simulink model "VehicleDynamicsModel"  (R2018a)
settings: Solver=ode15s  StartTime=0.0  StopTime=12  FixedStep=0.01  RelTol=1e-2  EnableMultiTasking=on
PreLoadFcn:
  | PowerTrain_14DOF_ini
StopFcn:
  | AfterSim
undefined symbols (not defined in the file): AccelCmd2TrqCmd, Chasis, GearRatio, Motor, Motor_J, Motor_RotorDamping, VEH, X, Y, Z
libraries: sm_lib x186, autolibutils x40, nesl_utility x23, vehdynlibtire x4, fuzblock x3, sharedtransform x2, autolibmappedmotorcommon x2, vehdynlibeom x1, vehdynlibsuspension x1, simulink x1, vehdynlibsteering x1
(part 1 of 11)
settings Model: SimulationMode=accelerator  ExtModeTrigDuration=100  Creator=rjackey  LastModifiedBy=Administrator
settings DataIOCC: ExternalInput=[Throttle.Time Throttle.Data Brake.Data]  LimitDataPoints=on  SaveFormat=StructureWithTime  SaveOutput=off  DSMLogging=off  SaveTime=off  StateSaveName=tmp_raccel_xout  OutputSaveName=out
settings OptimizationCC: DefaultUnderspecifiedDataType=single  ExpressionDepthLimit=2147483647  EfficientMapNaN2IntZero=off  LifeSpan=inf
settings DebuggingCC: UnderspecifiedInitializationDetection=Classic  MergeDetectMultiDrivingBlocksExec=none  SolverPrmCheckMsg=warning  UnnecessaryDatatypeConvMsg=warning  FcnCallInpInsideContextMsg=warning  StateNameClashWarn=warning  SFUnexpectedBacktrackingDiag=warning  SFNoUnconditionalDefaultTransitionDiag=warning  SFExecutionAtInitializationDiag=none
settings HardwareCC: ProdBitPerPointer=32  ProdBitPerSizeT=32  ProdBitPerPtrDiffT=32  ProdLargestAtomicFloat=None  ProdIntDivRoundTo=Undefined  ProdEndianess=Unspecified  ProdWordSize=32  ProdHWDeviceType=32-bit Generic  TargetBitPerPointer=64  TargetBitPerSizeT=64  TargetBitPerPtrDiffT=64  TargetLongLongMode=on  TargetIntDivRoundTo=Zero  TargetEndianess=LittleEndian  TargetWordSize=64  TargetHWDeviceType=MATLAB Host  ProdEqTarget=off
settings ModelReferenceCC: PropagateSignalLabelsOutOfModel=off
settings RTWCC: SystemTargetFile=raccel.tlc  TemplateMakefile=raccel_default_tmf  RTWVerbose=off  RTWUseSimCustomCode=on
settings CodeAppCC: GenerateComments=off  MaxIdLength=128  MangleLength=10
settings RaccelTargetCC: GeneratePreprocessorConditionals=Use local settings  MultiInstanceERTCode=off  ENABLE_SLEXEC_SSBRIDGE=1  RTWCAPIParams=on
settings ConfigComp: CovScope=ReferencedModels  CovIncludeTopModel=off  CovMetricSettings=dw  CovHtmlReporting=on  CovSaveCumulativeToWorkspaceVar=on  CovSaveSingleToWorkspaceVar=on  CovExternalEMLEnable=off
settings SimscapeCC: SimscapeNormalizeSystem=off
settings ExplorerConfigSet: SimMechanicsOpenEditorOnUpdate=off

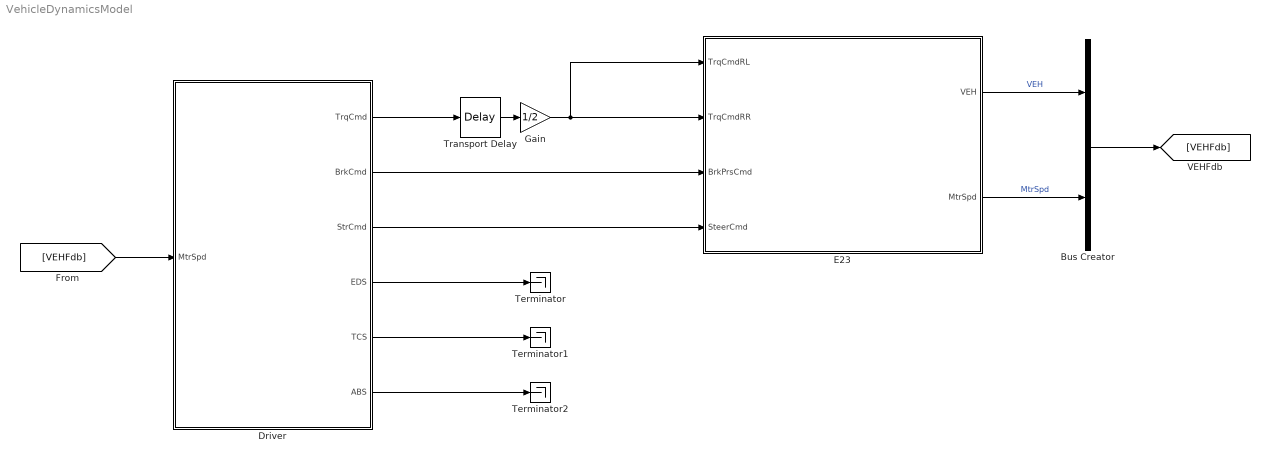
== system VehicleDynamicsModel ==
  Bus Creator : BusCreator  Inputs=2
  Driver : Subsystem
      mask Display: image('Driver.JPEG');
  E23 : Subsystem
      mask Display: image('E2314DOF2.jpg')
  Gain : Gain  Gain=1/2
  Terminator : Terminator
  Terminator1 : Terminator
  Terminator2 : Terminator
  Transport Delay : TransportDelay  DelayTime=0.1
  wires:
  Driver/3(StrCmd) -> E23/4(SteerCmd)
  Driver/2(BrkCmd) -> E23/3(BrkPrsCmd)
  E23/2(MtrSpd) -> Bus Creator/2  "MtrSpd"
  E23/1(VEH) -> Bus Creator/1  "VEH"
  Bus Creator/1 -> [VEHFdb]
  [VEHFdb] -> Driver/1(MtrSpd)
  Driver/1(TrqCmd) -> Transport Delay/1
  Gain/1 -> E23/2(TrqCmdRR), E23/1(TrqCmdRL)
  Transport Delay/1 -> Gain/1
  Driver/4(EDS) -> Terminator/1
  Driver/5(TCS) -> Terminator1/1
  Driver/6(ABS) -> Terminator2/1

== system VehicleDynamicsModel/Driver ==
  MtrSpd : Inport
  AccCmdGenerate : Subsystem
  Accel : Subsystem
  BrkCmdGenerate : Subsystem
  Bus Selector : BusSelector  OutputSignals=MtrSpd.MtrSpdRL,MtrSpd.MtrSpdRR
  Constant{1,5..7} (4 alike) : Constant  Value=0
  Mux : Mux
  Saturation : Saturate  UpperLimit=1  LowerLimit=0
  StrCmdGenerate : Subsystem
  Terminator3 : Terminator
  TrqCmd : Outport
  BrkCmd : Outport  Port=2
  StrCmd : Outport  Port=3
  EDS : Outport  Port=4
  TCS : Outport  Port=5
  ABS : Outport  Port=6
  wires:
  Saturation/1 -> Accel/3(AccelCmd)
  Constant5/1 -> EDS/1
  MtrSpd/1 -> Bus Selector/1
  Constant1/1 -> Mux/2, Mux/1, Mux/4, Mux/3
  Constant6/1 -> TCS/1
  Accel/1(TrqCmd) -> TrqCmd/1
  Constant7/1 -> ABS/1
  Bus Selector/2 -> Accel/2(MtrSpdRR)  "<MtrSpdRR>"
  Bus Selector/1 -> Accel/1(MtrSpdRL)  "<MtrSpdRL>"
  Mux/1 -> BrkCmd/1
  BrkCmdGenerate/1(BrkCmd) -> Terminator3/1  "BrkCmd"
  AccCmdGenerate/1(AccCmd) -> Saturation/1  "AccCmd"
  StrCmdGenerate/1(StrCmd) -> StrCmd/1  "StrCmd"

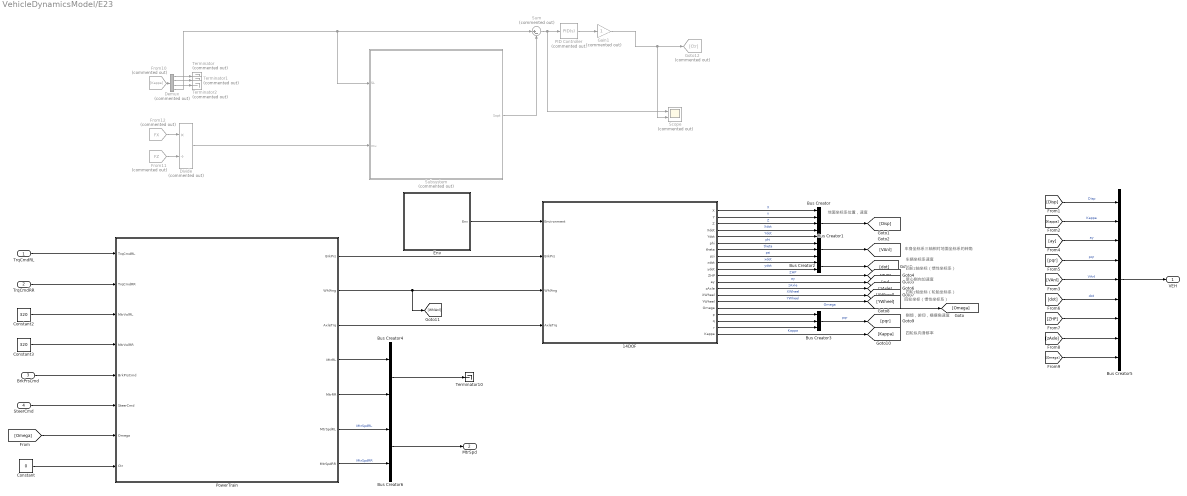
== system VehicleDynamicsModel/E23 ==
  note: 侧倾，俯仰，横摆角速度
  note: 四轮坐标（惯性坐标系）
  note: 质心侧向加速度
  note: 四轮z轴坐标（惯性坐标系）
  note: 车身坐标系三轴相对地面坐标系的转角
  note: 地面坐标系位置，速度
  note: 车辆坐标系速度
  note: 四轮z轴坐标（轮胎坐标系）
  note: 四轮纵向滑移率
  TrqCmdRL : Inport
  TrqCmdRR : Inport  Port=2
  BrkPrsCmd : Inport  Port=3
  SteerCmd : Inport  Port=4
  14DOF : Subsystem
      mask Display: image('E2314DOF.jpg')
  Bus Creator : BusCreator  Inputs=5
  Bus Creator1 : BusCreator  Inputs=3
  Bus Creator2 : BusCreator  Inputs=2
  Bus Creator3 : BusCreator  Inputs=3
  Bus Creator4 : BusCreator  Inputs=2
  Bus Creator5 : BusCreator  Inputs=9
  Bus Creator6 : BusCreator  Inputs=2
  Constant : Constant  Value=0
  Constant2 : Constant  Value=320
  Constant3 : Constant  Value=320
  Demux : Demux  Commented=on
  Divide : Product  Commented=on  Inputs=*/
  Env : Subsystem
      mask Display: image('Env.jpg')
  From10 : From  Commented=on  GotoTag=Kappa
  From11 : From  Commented=on  GotoTag=FZ  TagVisibility=global
  From12 : From  Commented=on  GotoTag=FX  TagVisibility=global
  Gain1 : Gain  Commented=on
  Goto12 : Goto  Commented=on  GotoTag=Ctr
  PID Controller : simulink/Continuous/PID Controller  Commented=on  Controller=PID  TimeDomain=Continuous-time  SampleTime=-1  IntegratorMethod=Forward Euler  FilterMethod=Forward Euler  Form=Parallel  UseFilter=on  ControllerParametersSource=internal  P=500  I=20  D=0  N=100  InitialConditionSource=internal  InitialConditionForIntegrator=0  InitialConditionForFilter=0  ExternalReset=none  LimitOutput=off  UpperSaturationLimit=inf  LowerSaturationLimit=-inf  LinearizeAsGain=on  AntiWindupMode=none  Kb=1  TrackingMode=off  Kt=1  PParamMin=[]  PParamMax=[]  IParamMin=[]  IParamMax=[]  DParamMin=[]  DParamMax=[]  NParamMin=[]  NParamMax=[]  KbParamMin=[]  KbParamMax=[]  KtParamMin=[]  KtParamMax=[]  POutMin=[]  POutMax=[]  IOutMin=[]  IOutMax=[]  DOutMin=[]  DOutMax=[]  NOutMin=[]  NOutMax=[]  KbOutMin=[]  KbOutMax=[]  KtOutMin=[]  KtOutMax=[]  IntegratorOutMin=[]  IntegratorOutMax=[]  FilterOutMin=[]  FilterOutMax=[]  SumOutMin=[]  SumOutMax=[]  SumI1OutMin=[]  SumI1OutMax=[]  SumI2OutMin=[]  SumI2OutMax=[]  SumI3OutMin=[]  SumI3OutMax=[]  SumDOutMin=[]  SumDOutMax=[]  SaturationOutMin=[]  SaturationOutMax=[]  IntegratorContinuousStateAttributes=''  IntegratorStateMustResolveToSignalObject=off  IntegratorRTWStateStorageClass=Auto  FilterContinuousStateAttributes=''  FilterStateMustResolveToSignalObject=off  FilterRTWStateStorageClass=Auto  DifferentiatorICPrevScaledInput=0  DifferentiatorOutMin=[]  DifferentiatorOutMax=[]  FilterDiffOutCoefMin=[]  FilterDiffOutCoefMax=[]  SumDenOutMin=[]  SumDenOutMax=[]  SumNumOutMin=[]  SumNumOutMax=[]  ReciprocalOutMin=[]  ReciprocalOutMax=[]  DivideOutMin=[]  DivideOutMax=[]  TunerSelectOption=Transfer Function Based (PID Tuner App)
  PowerTrain : Subsystem
      mask Display: image('PowerTrain.jpg')
  Scope : Scope  Commented=on  NumInputPorts=2
  Subsystem : Subsystem  Commented=on
  Sum : Sum  Commented=on  Inputs=|+-
  Terminator : Terminator  Commented=on
  Terminator1 : Terminator  Commented=on
  Terminator10 : Terminator
  Terminator2 : Terminator  Commented=on
  VEH : Outport
  MtrSpd : Outport  Port=2
  wires:
  Bus Creator3/1 -> [pqr]  "pqr"
  14DOF/20(Kappa) -> [Kappa]  "Kappa"
  14DOF/15(YWheel) -> [YWheel]  "YWheel"
  14DOF/9(xdot) -> Bus Creator2/1  "xdot"
  [VAnl] -> Bus Creator5/5  "VAnl"
  PowerTrain/3(AxleTrq) -> 14DOF/4(AxleTrq)
  Bus Creator1/1 -> [VAnl]
  Bus Creator5/1 -> VEH/1
  14DOF/18(q) -> Bus Creator3/2
  Bus Creator/1 -> [Disp]
  [dot] -> Bus Creator5/6  "dot"
  14DOF/12(ay) -> [ay]  "ay"
  [pqr] -> Bus Creator5/4  "pqr"
  Bus Creator2/1 -> [dot]
  14DOF/14(XWheel) -> [XWheel]  "XWheel"
  PowerTrain/2(WhlAng) -> [WhlAnl], 14DOF/3(WhlAng)
  14DOF/11(ZHP) -> [ZHP]  "ZHP"
  TrqCmdRR/1 -> PowerTrain/2(TrqCmdRR)
  14DOF/7(theta) -> Bus Creator1/2  "theta"
  14DOF/16(Omega) -> [Omega]  "Omega"
  14DOF/1(X) -> Bus Creator/1  "X"
  14DOF/19(r) -> Bus Creator3/3
  Env/1(Env) -> 14DOF/1(Environment)
  14DOF/17(p) -> Bus Creator3/1
  14DOF/2(Y) -> Bus Creator/2  "Y"
  14DOF/3(Z) -> Bus Creator/3  "Z"
  [Disp] -> Bus Creator5/1  "Disp"
  PowerTrain/1(BrkPrs) -> 14DOF/2(BrkPrs)
  14DOF/5(Ydot) -> Bus Creator/5  "Ydot"
  14DOF/4(Xdot) -> Bus Creator/4  "Xdot"
  14DOF/6(phi) -> Bus Creator1/1  "phi"
  14DOF/10(ydot) -> Bus Creator2/2  "ydot"
  SteerCmd/1 -> PowerTrain/6(SteerCmd)
  PowerTrain/4(MtrRL) -> Bus Creator4/1
  Bus Creator4/1 -> Terminator10/1
  TrqCmdRL/1 -> PowerTrain/1(TrqCmdRL)
  Constant2/1 -> PowerTrain/3(MtrVolRL)
  Constant3/1 -> PowerTrain/4(MtrVolRR)
  BrkPrsCmd/1 -> PowerTrain/5(BrkPrsCmd)
  PowerTrain/5(MtrRR) -> Bus Creator4/2
  14DOF/8(psi) -> Bus Creator1/3  "psi"
  [Omega] -> PowerTrain/7(Omega)
  [Kappa] -> Bus Creator5/2  "Kappa"
  [ay] -> Bus Creator5/3  "ay"
  14DOF/13(zAxle) -> [zAxle]  "zAxle"
  [ZHP] -> Bus Creator5/7
  [zAxle] -> Bus Creator5/8
  [Omega] -> Bus Creator5/9
  PowerTrain/6(MtrSpdRL) -> Bus Creator6/1  "MtrSpdRL"
  PowerTrain/7(MtrSpdRR) -> Bus Creator6/2  "MtrSpdRR"
  Bus Creator6/1 -> MtrSpd/1
  Demux/4 -> Subsystem/1(SL), Sum/1
  Gain1/1 -> Scope/2, Goto12/1
  Subsystem/1(Sopt) -> Sum/2
  Sum/1 -> Scope/1, PID Controller/1
  Divide/1 -> Subsystem/2(mu)
  PID Controller/1 -> Gain1/1
  From10/1 -> Demux/1
  Demux/1 -> Terminator/1
  Demux/2 -> Terminator1/1
  Demux/3 -> Terminator2/1
  From12/1 -> Divide/1
  From11/1 -> Divide/2
  Constant/1 -> PowerTrain/8(Ctr)

== system VehicleDynamicsModel/Driver/AccCmdGenerate ==
  Clock : Clock
  Constant : Constant
  Constant1 : Constant  Value=0
  Constant2 : Constant  Value=0.1
  Switch : Switch  Criteria=u2 > Threshold  Threshold=4
  Switch1 : Switch  Criteria=u2 > Threshold  Threshold=8
  AccCmd : Outport
  wires:
  Constant1/1 -> Switch/1
  Switch1/1 -> AccCmd/1
  Clock/1 -> Switch1/2, Switch/2
  Constant2/1 -> Switch1/1
  Switch/1 -> Switch1/3
  Constant/1 -> Switch/3

== system VehicleDynamicsModel/Driver/Accel ==
  MtrSpdRL : Inport
  MtrSpdRR : Inport  Port=2
  AccelCmd : Inport  Port=3
  Add : Sum
  LookupTable : Lookup_n-D  BreakpointsForDimension1=AccelCmd2TrqCmd.Motor_n  BreakpointsForDimension2=fliplr(AccelCmd2TrqCmd.AccelCmd)  Table=fliplr(AccelCmd2TrqCmd.TrqCmd)  InternalRulePriority=Speed  RndMeth=Simplest  InputSameDT=on
  LookupTable1 : Lookup_n-D  BreakpointsForDimension1=AccelCmd2TrqCmd.Motor_n  BreakpointsForDimension2=fliplr(AccelCmd2TrqCmd.AccelCmd)  Table=fliplr(AccelCmd2TrqCmd.TrqCmd)  InternalRulePriority=Speed  RndMeth=Simplest  InputSameDT=on
  TrqCmd : Outport
  wires:
  LookupTable/1 -> Add/1
  MtrSpdRL/1 -> LookupTable/1
  MtrSpdRR/1 -> LookupTable1/1
  AccelCmd/1 -> LookupTable1/2, LookupTable/2
  LookupTable1/1 -> Add/2
  Add/1 -> TrqCmd/1

== system VehicleDynamicsModel/Driver/BrkCmdGenerate ==
  Clock : Clock
  Constant : Constant  Value=0
  Constant1 : Constant  Value=0.6
  Constant2 : Constant  Value=0
  Switch : Switch  Criteria=u2 > Threshold  Threshold=5
  Switch1 : Switch  Criteria=u2 > Threshold  Threshold=5.5
  BrkCmd : Outport
  wires:
  Constant/1 -> Switch/3
  Switch/1 -> Switch1/3
  Constant2/1 -> Switch1/1
  Clock/1 -> Switch/2, Switch1/2
  Switch1/1 -> BrkCmd/1
  Constant1/1 -> Switch/1

== system VehicleDynamicsModel/Driver/StrCmdGenerate ==
  Sine Wave : Sin  Amplitude=0.6  Frequency=3.1415926/3  SampleTime=0
  Transport Delay : TransportDelay  DelayTime=6
  StrCmd : Outport
  wires:
  Transport Delay/1 -> StrCmd/1
  Sine Wave/1 -> Transport Delay/1

== system VehicleDynamicsModel/E23/14DOF ==
  note: 双电机后驱
  Environment : Inport
  BrkPrs : Inport  Port=2
  WhlAng : Inport  Port=3
  AxleTrq : Inport  Port=4
  14DOF : Subsystem
      mask Display: image('E2314DOF2.jpg')
  Bus Creator : BusCreator  Inputs=4
  Bus Selector : BusSelector  OutputSignals=Wind,Gnd,mu
  Bus Selector2 : BusSelector  OutputSignals=p,q,r
  Demux : Demux
  X : Outport
  Y : Outport  Port=2
  Z : Outport  Port=3
  Xdot : Outport  Port=4
  Ydot : Outport  Port=5
  phi : Outport  Port=6
  theta : Outport  Port=7
  psi : Outport  Port=8
  xdot : Outport  Port=9
  ydot : Outport  Port=10
  ZHP : Outport  Port=11
  ay : Outport  Port=12
  zAxle : Outport  Port=13
  XWheel : Outport  Port=14
  YWheel : Outport  Port=15
  Omega : Outport  Port=16
  p : Outport  Port=17
  q : Outport  Port=18
  r : Outport  Port=19
  Kappa : Outport  Port=20
  wires:
  14DOF/7(theta) -> theta/1
  Bus Creator/1 -> Omega/1
  Demux/3 -> Bus Creator/3  "OmegaRL"
  14DOF/10(ydot) -> ydot/1
  Demux/1 -> Bus Creator/1  "OmegaFL"
  14DOF/11(pqr) -> Bus Selector2/1
  14DOF/5(Ydot) -> Ydot/1
  Bus Selector2/1 -> p/1  "<p>"
  [Omega] -> Demux/1
  Demux/4 -> Bus Creator/4  "OmegaRR"
  Bus Selector/3 -> 14DOF/6(Friction)  "<mu>"
  Bus Selector2/3 -> r/1  "<r>"
  Bus Selector/1 -> 14DOF/4(Wind)  "<Wind>"
  14DOF/8(psi) -> psi/1
  14DOF/18(YWheel) -> YWheel/1
  14DOF/6(phi) -> phi/1
  Bus Selector/2 -> 14DOF/5(GroundXYZ)  "<Gnd>"
  14DOF/16(kappa) -> Kappa/1
  Bus Selector2/2 -> q/1  "<q>"
  14DOF/17(XWheel) -> XWheel/1
  14DOF/13(ay) -> ay/1
  14DOF/14(omega) -> [Omega]
  Demux/2 -> Bus Creator/2  "OmegaFR"
  14DOF/12(ZHP) -> ZHP/1
  14DOF/3(Z) -> Z/1
  14DOF/15(zAxle) -> zAxle/1
  14DOF/2(Y) -> Y/1
  14DOF/9(xdot) -> xdot/1
  14DOF/1(X) -> X/1
  Environment/1 -> Bus Selector/1
  BrkPrs/1 -> 14DOF/2(BrkPrs)
  WhlAng/1 -> 14DOF/3(WheelAngle)
  AxleTrq/1 -> 14DOF/1(AxleTrq)
  14DOF/4(Xdot) -> Xdot/1

== system VehicleDynamicsModel/E23/Env ==
  note: 峰值附着系数
  Bus Creator : BusCreator  Inputs=4
  Bus Creator1 : BusCreator  Inputs=3
  Bus Creator2 : BusCreator  Inputs=4
  Constant3 : Constant  Value=0
  Constant7 : Constant  Value=zeros(4,1)
  Demux : Demux
  Demux1 : Demux
  Friction : Constant  Value=1.4*ones(4,1)
  Vector Concatenate3 : Concatenate  NumInputs=3
  Env : Outport
  wires:
  Constant3/1 -> Vector Concatenate3/3, Vector Concatenate3/2, Vector Concatenate3/1
  Demux1/2 -> Bus Creator2/2  "mu_FR"
  Demux1/1 -> Bus Creator2/1  "mu_FL"
  Bus Creator/1 -> Bus Creator1/2  "Gnd"
  Demux/4 -> Bus Creator/4  "G_RR_z"
  Demux/3 -> Bus Creator/3  "G_RL_z"
  Vector Concatenate3/1 -> Bus Creator1/1  "Wind"
  Constant7/1 -> Demux/1
  Demux1/3 -> Bus Creator2/3  "mu_RL"
  Bus Creator2/1 -> Bus Creator1/3  "mu"
  Friction/1 -> Demux1/1
  Demux1/4 -> Bus Creator2/4  "mu_RR"
  Demux/2 -> Bus Creator/2  "G_FR_z"
  Demux/1 -> Bus Creator/1  "G_FL_z"
  Bus Creator1/1 -> Env/1

== system VehicleDynamicsModel/E23/PowerTrain ==
  TrqCmdRL : Inport
  TrqCmdRR : Inport  Port=2
  MtrVolRL : Inport  Port=3
  MtrVolRR : Inport  Port=4
  BrkPrsCmd : Inport  Port=5
  SteerCmd : Inport  Port=6
  Omega : Inport  Port=7
  Ctr : Inport  Port=8
  Bus Creator : BusCreator  Inputs=2
  Bus Creator1 : BusCreator  Inputs=2
  DriveTrain : Subsystem
  PowerTrain : Subsystem
  BrkPrs : Outport
  WhlAng : Outport  Port=2
  AxleTrq : Outport  Port=3
  MtrRL : Outport  Port=4
  MtrRR : Outport  Port=5
  MtrSpdRL : Outport  Port=6
  MtrSpdRR : Outport  Port=7
  wires:
  PowerTrain/5(MtrTrqRL) -> DriveTrain/3(MtrTrqRL)
  DriveTrain/3(AxleTrq) -> AxleTrq/1
  PowerTrain/1(MechPwrRL) -> Bus Creator/1
  PowerTrain/2(EfficiencyRL) -> Bus Creator/2
  TrqCmdRR/1 -> PowerTrain/2(TrqCmdRR)
  PowerTrain/6(MtrTrqRR) -> DriveTrain/4(MtrTrqRR)
  DriveTrain/1(BrkPrs) -> BrkPrs/1
  TrqCmdRL/1 -> PowerTrain/1(TrqCmdRL)
  DriveTrain/2(WhlAng) -> WhlAng/1
  PowerTrain/3(MechPwrRR) -> Bus Creator1/1
  MtrVolRR/1 -> PowerTrain/4(MtrVolRR)
  PowerTrain/4(EfficiencyRR) -> Bus Creator1/2
  MtrVolRL/1 -> PowerTrain/3(MtrVolRL)
  Bus Creator1/1 -> MtrRR/1
  Bus Creator/1 -> MtrRL/1
  SteerCmd/1 -> DriveTrain/2(SteerCmd)
  BrkPrsCmd/1 -> DriveTrain/1(BrkPrsCmd)
  Omega/1 -> PowerTrain/5(Omega)
  PowerTrain/8(MtrSpdRR) -> MtrSpdRR/1
  PowerTrain/7(MtrSpdRL) -> MtrSpdRL/1
  Ctr/1 -> PowerTrain/6(Ctr)

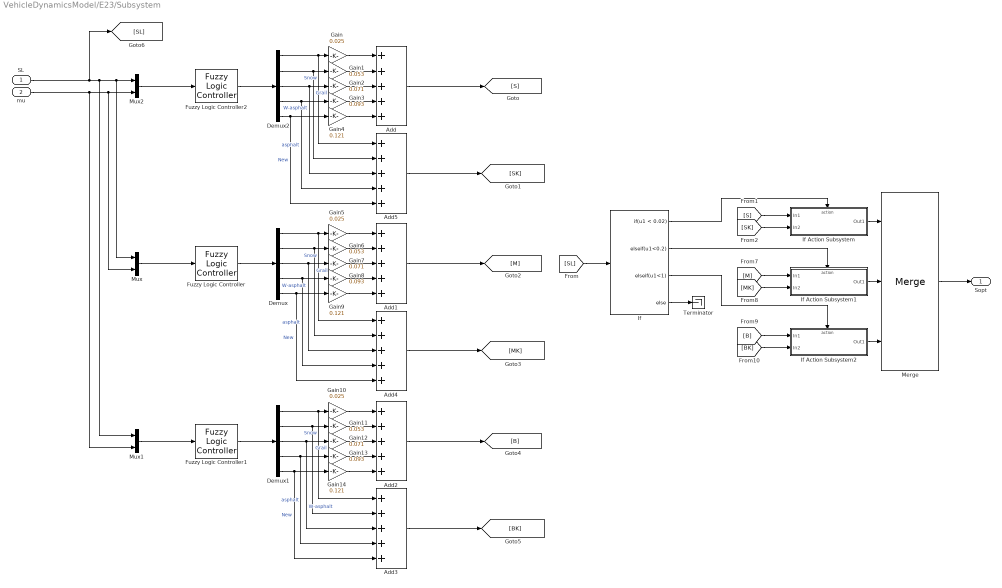
== system VehicleDynamicsModel/E23/Subsystem ==
  SL : Inport
  mu : Inport  Port=2
  Add{,1..5} (6 alike) : Sum  Inputs=+++++
  Demux : Demux  Outputs=5
  Demux1 : Demux  Outputs=5
  Demux2 : Demux  Outputs=5
  Fuzzy Logic Controller : fuzblock/Fuzzy Logic  Controller  FIS='FuzzyTCSM.fis'  OutputSampleNumber=101  DataType=double  FuzzifiedInputs=off  RuleFiringStrengths=off  RuleOutputs=off  AggregatedOutputs=off  SimulateUsing=Interpreted execution  OutOfRangeInputValueMessage=warning  NoRuleFiredMessage=warning  EmptyOutputFuzzySetMessage=warning
  Fuzzy Logic Controller1 : fuzblock/Fuzzy Logic  Controller  FIS='FuzzyTCSB.fis'  OutputSampleNumber=101  DataType=double  FuzzifiedInputs=off  RuleFiringStrengths=off  RuleOutputs=off  AggregatedOutputs=off  SimulateUsing=Interpreted execution  OutOfRangeInputValueMessage=warning  NoRuleFiredMessage=warning  EmptyOutputFuzzySetMessage=warning
  Fuzzy Logic Controller2 : fuzblock/Fuzzy Logic  Controller  FIS='FuzzyTCSS.fis'  OutputSampleNumber=101  DataType=double  FuzzifiedInputs=off  RuleFiringStrengths=off  RuleOutputs=off  AggregatedOutputs=off  SimulateUsing=Interpreted execution  OutOfRangeInputValueMessage=warning  NoRuleFiredMessage=warning  EmptyOutputFuzzySetMessage=warning
  Gain : Gain  Gain=0.025
  Gain1 : Gain  Gain=0.053
  Gain10 : Gain  Gain=0.025
  Gain11 : Gain  Gain=0.053
  Gain12 : Gain  Gain=0.071
  Gain13 : Gain  Gain=0.093
  Gain14 : Gain  Gain=0.121
  Gain2 : Gain  Gain=0.071
  Gain3 : Gain  Gain=0.093
  Gain4 : Gain  Gain=0.121
  Gain5 : Gain  Gain=0.025
  Gain6 : Gain  Gain=0.053
  Gain7 : Gain  Gain=0.071
  Gain8 : Gain  Gain=0.093
  Gain9 : Gain  Gain=0.121
  If : If  IfExpression=u1 < 0.02  ElseIfExpressions=u1<0.2,u1<1
  If Action Subsystem : Subsystem  TreatAsAtomicUnit=on
  If Action Subsystem1 : Subsystem  TreatAsAtomicUnit=on
  If Action Subsystem2 : Subsystem  TreatAsAtomicUnit=on
  Merge : Merge  Inputs=3
  Mux : Mux  Inputs=2
  Mux1 : Mux  Inputs=2
  Mux2 : Mux  Inputs=2
  Terminator : Terminator
  Sopt : Outport
  wires:
  Demux1/2 -> Add3/2, Gain11/1  "Grail"
  Gain8/1 -> Add1/4
  Add1/1 -> [M]
  Add4/1 -> [MK]
  SL/1 -> [SL], Mux1/1, Mux/1, Mux2/1
  Demux/5 -> Add4/5, Gain9/1  "New"
  Demux1/5 -> Add3/5, Gain14/1  "New"
  Gain/1 -> Add/1
  Gain7/1 -> Add1/3
  Add5/1 -> [SK]
  Demux2/4 -> Add5/4, Gain3/1  "asphalt"
  Demux2/5 -> Add5/5, Gain4/1  "New"
  Mux1/1 -> Fuzzy Logic Controller1/1
  Demux1/3 -> Add3/3, Gain12/1  "W-asphalt"
  Gain5/1 -> Add1/1
  Gain1/1 -> Add/2
  Gain9/1 -> Add1/5
  Demux1/4 -> Add3/4, Gain13/1  "asphalt"
  Demux/4 -> Add4/4, Gain8/1  "asphalt"
  Gain14/1 -> Add2/5
  Mux/1 -> Fuzzy Logic Controller/1
  Fuzzy Logic Controller2/1 -> Demux2/1
  Gain12/1 -> Add2/3
  Add3/1 -> [BK]
  mu/1 -> Mux1/2, Mux/2, Mux2/2
  Add2/1 -> [B]
  Add/1 -> [S]
  Gain3/1 -> Add/4
  Mux2/1 -> Fuzzy Logic Controller2/1
  Fuzzy Logic Controller1/1 -> Demux1/1
  Demux2/3 -> Add5/3, Gain2/1  "W-asphalt"
  Demux1/1 -> Add3/1, Gain10/1  "Snow"
  Gain10/1 -> Add2/1
  Demux/3 -> Add4/3, Gain7/1  "W-asphalt"
  Gain11/1 -> Add2/2
  Demux2/1 -> Add5/1, Gain/1  "Snow"
  Gain13/1 -> Add2/4
  Demux/1 -> Add4/1, Gain5/1  "Snow"
  Demux/2 -> Add4/2, Gain6/1  "Grail"
  Gain2/1 -> Add/3
  Demux2/2 -> Add5/2, Gain1/1  "Grail"
  Gain4/1 -> Add/5
  Fuzzy Logic Controller/1 -> Demux/1
  Gain6/1 -> Add1/2
  [SL] -> If/1
  [S] -> If Action Subsystem/1(In1)
  [SK] -> If Action Subsystem/2(In2)
  [M] -> If Action Subsystem1/1(In1)
  [MK] -> If Action Subsystem1/2(In2)
  [B] -> If Action Subsystem2/1(In1)
  [BK] -> If Action Subsystem2/2(In2)
  If/1 -> If Action Subsystem/Action
  If/2 -> If Action Subsystem1/Action
  If/3 -> If Action Subsystem2/Action
  If/4 -> Terminator/1
  Merge/1 -> Sopt/1
  If Action Subsystem/1(Out1) -> Merge/1
  If Action Subsystem1/1(Out1) -> Merge/2
  If Action Subsystem2/1(Out1) -> Merge/3

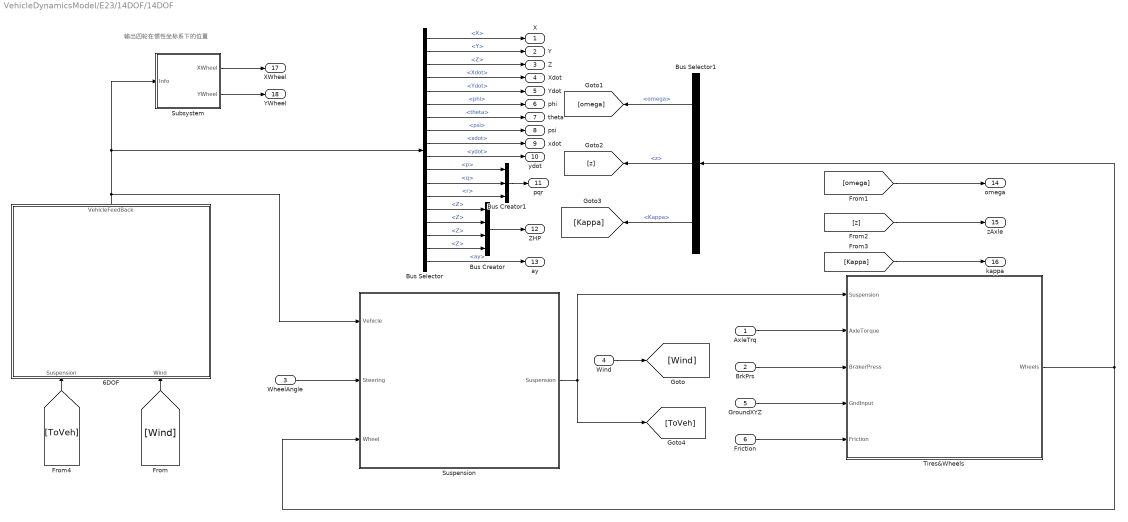
== system VehicleDynamicsModel/E23/14DOF/14DOF ==
  note: 输出四轮在惯性坐标系下的位置
  AxleTrq : Inport
  BrkPrs : Inport  Port=2
  WheelAngle : Inport  Port=3
  Wind : Inport  Port=4
  GroundXYZ : Inport  Port=5
  Friction : Inport  Port=6
  6DOF : Subsystem
      mask Display: image('E23.jpg');
  Bus Creator : BusCreator  Inputs=4
  Bus Creator1 : BusCreator  Inputs=3
  Bus Selector : BusSelector  OutputSignals=InertFrm.Cg.Disp.X,InertFrm.Cg.Disp.Y,InertFrm.Cg.Disp.Z,InertFrm.Cg.Vel.Xdot,InertFrm.Cg.Vel.Ydot,InertFrm.Cg.Ang.phi,InertFrm.Cg.Ang.theta,InertFrm.Cg.Ang.psi,BdyFrm.Cg.Vel.xdot,BdyFrm.Cg.Vel.ydot,BdyFrm.Cg.AngVel.p,BdyFrm.Cg.AngVel.q,BdyFrm.Cg.AngVel.r,InertFrm.FrntAxl.Lft.Disp.Z,InertFrm.FrntAxl.Rght.Disp.Z,InertFrm.RearAxl.Lft.Disp.Z,InertFrm.RearAxl.Rght.Disp.Z,BdyFrm.Cg.Acc.ay
  Bus Selector1 : BusSelector  OutputSignals=TireFrame.omega,TireFrame.z,TireFrame.Kappa
  Subsystem : Subsystem
  Suspension : Subsystem
      mask Display: image('Suspen.jpg');
  Tires&Wheels : Subsystem
      mask Display: image('WheelsTires.jpg');
  X : Outport
  Y : Outport  Port=2
  Z : Outport  Port=3
  Xdot : Outport  Port=4
  Ydot : Outport  Port=5
  phi : Outport  Port=6
  theta : Outport  Port=7
  psi : Outport  Port=8
  xdot : Outport  Port=9
  ydot : Outport  Port=10
  pqr : Outport  Port=11
  ZHP : Outport  Port=12
  ay : Outport  Port=13
  omega : Outport  Port=14
  zAxle : Outport  Port=15
  kappa : Outport  Port=16
  XWheel : Outport  Port=17
  YWheel : Outport  Port=18
  wires:
  Bus Selector/6 -> phi/1  "<phi>"
  Suspension/1(Suspension) -> Tires&Wheels/1(Suspension), [ToVeh]
  BrkPrs/1 -> Tires&Wheels/3(BrakerPress)
  Bus Selector/5 -> Ydot/1  "<Ydot>"
  Bus Selector/9 -> xdot/1  "<xdot>"
  Bus Selector1/3 -> [Kappa]  "<Kappa>"
  Bus Selector/16 -> Bus Creator/3  "<Z>"
  Bus Selector/7 -> theta/1  "<theta>"
  GroundXYZ/1 -> Tires&Wheels/4(GndInput)
  Bus Selector/17 -> Bus Creator/4  "<Z>"
  Bus Selector/1 -> X/1  "<X>"
  Bus Selector/2 -> Y/1  "<Y>"
  Subsystem/1(XWheel) -> XWheel/1
  AxleTrq/1 -> Tires&Wheels/2(AxleTorque)
  Bus Selector/15 -> Bus Creator/2  "<Z>"
  Bus Selector1/2 -> [z]  "<z>"
  Bus Selector/14 -> Bus Creator/1  "<Z>"
  Bus Selector/10 -> ydot/1  "<ydot>"
  [Wind] -> 6DOF/2(Wind)
  6DOF/1(VehicleFeedBack) -> Suspension/1(Vehicle), Bus Selector/1, Subsystem/1(Info)
  Bus Selector/3 -> Z/1  "<Z>"
  Bus Creator/1 -> ZHP/1
  Friction/1 -> Tires&Wheels/5(Friction)
  Bus Selector/8 -> psi/1  "<psi>"
  Bus Selector/18 -> ay/1  "<ay>"
  Subsystem/2(YWheel) -> YWheel/1
  Bus Selector/4 -> Xdot/1  "<Xdot>"
  Bus Selector1/1 -> [omega]  "<omega>"
  WheelAngle/1 -> Suspension/2(Steering)
  Wind/1 -> [Wind]
  [omega] -> omega/1
  [z] -> zAxle/1
  [Kappa] -> kappa/1
  [ToVeh] -> 6DOF/1(Suspension)
  Tires&Wheels/1(Wheels) -> Suspension/3(Wheel), Bus Selector1/1
  Bus Selector/11 -> Bus Creator1/1  "<p>"
  Bus Selector/12 -> Bus Creator1/2  "<q>"
  Bus Selector/13 -> Bus Creator1/3  "<r>"
  Bus Creator1/1 -> pqr/1

== system VehicleDynamicsModel/E23/PowerTrain/DriveTrain ==
  BrkPrsCmd : Inport
  SteerCmd : Inport  Port=2
  MtrTrqRL : Inport  Port=3
  MtrTrqRR : Inport  Port=4
  DriveLine : Subsystem
  MotorTrq2AxleTrq : Subsystem
  BrkPrs : Outport
  WhlAng : Outport  Port=2
  AxleTrq : Outport  Port=3
  wires:
  DriveLine/1(AxleTrq) -> AxleTrq/1
  BrkPrsCmd/1 -> [BrkPrsCmd]
  DriveLine/3(WhlAng) -> WhlAng/1
  [SteerCmd] -> DriveLine/1(SteerCmd)
  SteerCmd/1 -> [SteerCmd]
  [BrkPrsCmd] -> DriveLine/3(BrkPrsCmd)
  DriveLine/2(BrakePressure) -> BrkPrs/1
  MtrTrqRL/1 -> MotorTrq2AxleTrq/1(MotorRL)
  MtrTrqRR/1 -> MotorTrq2AxleTrq/2(MotorRR)
  MotorTrq2AxleTrq/1(AxleTrq) -> DriveLine/2(AxleTrqCmd)

== system VehicleDynamicsModel/E23/PowerTrain/PowerTrain ==
  TrqCmdRL : Inport
  TrqCmdRR : Inport  Port=2
  MtrVolRL : Inport  Port=3
  MtrVolRR : Inport  Port=4
  Omega : Inport  Port=5
  Ctr : Inport  Port=6
  Bus Selector1 : BusSelector  OutputSignals=OmegaRL,OmegaRR
  Gain1 : Gain  Gain=GearRatio
  Gain2 : Gain  Gain=GearRatio
  MotorRL : Subsystem
      mask Display: image('Motor.jpg');
  MotorRR : Subsystem
      mask Display: image('Motor.jpg');
  Saturation : Saturate  UpperLimit=120  LowerLimit=0
  Saturation1 : Saturate  UpperLimit=120  LowerLimit=0
  Sum : Sum  Inputs=|-+
  Sum1 : Sum  Inputs=|+-
  Transfer Fcn{,1..3} (4 alike) : TransferFcn  Denominator=[0.005 1]
  MechPwrRL : Outport
  EfficiencyRL : Outport  Port=2
  MechPwrRR : Outport  Port=3
  EfficiencyRR : Outport  Port=4
  MtrTrqRL : Outport  Port=5
  MtrTrqRR : Outport  Port=6
  MtrSpdRL : Outport  Port=7
  MtrSpdRR : Outport  Port=8
  wires:
  TrqCmdRL/1 -> Sum/2
  MotorRR/2(Efficiency) -> EfficiencyRR/1
  Bus Selector1/2 -> Transfer Fcn1/1  "<OmegaRR>"
  MotorRL/2(Efficiency) -> EfficiencyRL/1
  MotorRR/1(MechPwr) -> MechPwrRR/1
  Transfer Fcn/1 -> Gain2/1
  MotorRL/3(MtrTrq) -> Transfer Fcn2/1
  MtrVolRR/1 -> MotorRR/3(MtrVol)
  MotorRL/1(MechPwr) -> MechPwrRL/1
  Transfer Fcn2/1 -> MtrTrqRL/1
  Gain2/1 -> MotorRL/2(MtrSpd), MtrSpdRL/1
  Transfer Fcn3/1 -> MtrTrqRR/1
  Transfer Fcn1/1 -> Gain1/1
  [OmegaRAxle] -> Bus Selector1/1
  Bus Selector1/1 -> Transfer Fcn/1  "<OmegaRL>"
  MotorRR/3(MtrTrq) -> Transfer Fcn3/1
  TrqCmdRR/1 -> Sum1/1
  MtrVolRL/1 -> MotorRL/3(MtrVol)
  Omega/1 -> [OmegaRAxle]
  Gain1/1 -> MotorRR/2(MtrSpd), MtrSpdRR/1
  Ctr/1 -> Sum1/2, Sum/1
  Saturation/1 -> MotorRL/1(TrqCmd)
  Saturation1/1 -> MotorRR/1(TrqCmd)
  Sum/1 -> Saturation/1
  Sum1/1 -> Saturation1/1

== system VehicleDynamicsModel/E23/Subsystem/If Action Subsystem ==
  In1 : Inport
  In2 : Inport  Port=2
  Action Port : ActionPort  ActionType=then
  Divide1 : Product  Inputs=*/
  Out1 : Outport
  wires:
  In2/1 -> Divide1/2
  Divide1/1 -> Out1/1
  In1/1 -> Divide1/1

== system VehicleDynamicsModel/E23/Subsystem/If Action Subsystem1 ==
  In1 : Inport
  In2 : Inport  Port=2
  Action Port : ActionPort  ActionType=elseif
  Divide1 : Product  Inputs=*/
  Out1 : Outport
  wires:
  In2/1 -> Divide1/2
  Divide1/1 -> Out1/1
  In1/1 -> Divide1/1

== system VehicleDynamicsModel/E23/Subsystem/If Action Subsystem2 ==
  In1 : Inport
  In2 : Inport  Port=2
  Action Port : ActionPort  ActionType=elseif
  Divide1 : Product  Inputs=*/
  Out1 : Outport
  wires:
  In2/1 -> Divide1/2
  Divide1/1 -> Out1/1
  In1/1 -> Divide1/1

== system VehicleDynamicsModel/E23/14DOF/14DOF/6DOF ==
  note: 外力，外力矩
  note: 质心在三个轴上的速度（惯性参考系）
  note: 质心在三个轴上的位置（惯性参考系）
  note: 欧拉角
  note: x，y，z轴的方向余弦
  note: 车身绕x，y，z轴的角速度（车身坐标系）
  note: 车辆质心在x，y，z轴上的速度分量（车身坐标系）
  Suspension : Inport
  Wind : Inport  Port=2
  Bus Selector : BusSelector  OutputSignals=Veh.F,Veh.M
  FExt : Constant  Value=[0;0;0]
  MExt : Constant  Value=[0;0;0]
  Scope : Scope  Commented=on  NumInputPorts=12
  Selector : Selector  Commented=on  NumberOfDimensions=2  InputPortWidth=3  IndexOptions=Index vector (dialog),Select all  Indices=1,1  OutputSizes=1,1
  Selector1 : Selector  Commented=on  NumberOfDimensions=2  InputPortWidth=3  IndexOptions=Index vector (dialog),Select all  Indices=2,1  OutputSizes=1,1
  Selector10 : Selector  Commented=on  InputPortWidth=4  IndexOptions=Index vector (dialog)  Indices=4  OutputSizes=1
  Selector11 : Selector  Commented=on  InputPortWidth=4  IndexOptions=Index vector (dialog)  Indices=4  OutputSizes=1
  Selector12 : Selector  Commented=on  InputPortWidth=4  IndexOptions=Index vector (dialog)  Indices=1  OutputSizes=1
  Selector13 : Selector  Commented=on  InputPortWidth=4  IndexOptions=Index vector (dialog)  Indices=2  OutputSizes=1
  Selector14 : Selector  Commented=on  InputPortWidth=4  IndexOptions=Index vector (dialog)  Indices=3  OutputSizes=1
  Selector2 : Selector  Commented=on  NumberOfDimensions=2  InputPortWidth=3  IndexOptions=Index vector (dialog),Select all  Indices=3,1  OutputSizes=1,1
  Selector3 : Selector  Commented=on  InputPortWidth=4  IndexOptions=Index vector (dialog)  Indices=1  OutputSizes=1
  Selector4 : Selector  Commented=on  InputPortWidth=4  IndexOptions=Index vector (dialog)  Indices=2  OutputSizes=1
  Selector5 : Selector  Commented=on  InputPortWidth=4  IndexOptions=Index vector (dialog)  Indices=3  OutputSizes=1
  Selector6 : Selector  Commented=on  InputPortWidth=4  IndexOptions=Index vector (dialog)  Indices=4  OutputSizes=1
  Selector7 : Selector  Commented=on  InputPortWidth=4  IndexOptions=Index vector (dialog)  Indices=1  OutputSizes=1
  Selector8 : Selector  Commented=on  InputPortWidth=4  IndexOptions=Index vector (dialog)  Indices=2  OutputSizes=1
  Selector9 : Selector  Commented=on  InputPortWidth=4  IndexOptions=Index vector (dialog)  Indices=3  OutputSizes=1
  Terminator{,1..5} (6 alike) : Terminator
  Vehicle Body 6DOF : vehdynlibeom/Vehicle Body 6DOF  m=VEH.Mass  a=VEH.FrontAxlePositionfromCG  b=VEH.RearAxlePositionfromCG  h=VEH.HeightCG  Xe_o=[VEH.InitialLongPosition,VEH.InitialLatPosition,VEH.InitialVertPosition]  xbdot_o=[VEH.InitialLongVel,VEH.InitialLatVel,VEH.InitialVertVel]  eul_o=[VEH.InitialRollAngle,VEH.InitialPitchAngle,VEH.InitialYawAngle]  p_o=[VEH.InitialRollRate,VEH.InitialPitchRate,VEH.InitialYawRate]  Iveh=[VEH.RollMomentInertia 0 0; 0 VEH.PitchMomentInertia 0; 0 0 VEH.YawMomentInertia]  w=VEH.TrackWidth.*[1 1]  Af=VEH.FrontalArea  Cd=.3  Cl=.1  Cpm=.1  beta_w=[0:0.01:0.3]  Cs=[0:0.03:0.9]  Cym=[0:0.01:0.3]  Pabs=101325  Tair=273  g=9.81  aMode=2
      settings: SourceProductName=Vehicle Dynamics Blockset  SourceProductBaseCode=VE
  VehicleFeedBack : Outport
  wires:
  MExt/1 -> Vehicle Body 6DOF/4
  Vehicle Body 6DOF/6 -> Terminator4/1
  Vehicle Body 6DOF/7 -> Terminator5/1
  Vehicle Body 6DOF/5 -> Terminator3/1
  Vehicle Body 6DOF/1 -> VehicleFeedBack/1
  FExt/1 -> Vehicle Body 6DOF/3
  Bus Selector/1 -> Selector/1, Selector1/1, Selector2/1, Vehicle Body 6DOF/1  "<F>"
  Suspension/1 -> Bus Selector/1
  Vehicle Body 6DOF/3 -> Terminator1/1
  Bus Selector/2 -> Vehicle Body 6DOF/2  "<M>"
  Wind/1 -> Vehicle Body 6DOF/5
  Vehicle Body 6DOF/2 -> Terminator/1
  Vehicle Body 6DOF/4 -> Terminator2/1
  Selector/1 -> Selector6/1, Selector5/1, Selector4/1, Selector3/1
  Selector1/1 -> Selector7/1, Selector8/1, Selector9/1, Selector10/1
  Selector2/1 -> Selector11/1, Selector14/1, Selector12/1, Selector13/1
  Selector3/1 -> Scope/1
  Selector4/1 -> Scope/2
  Selector5/1 -> Scope/3
  Selector6/1 -> Scope/4
  Selector7/1 -> Scope/5
  Selector8/1 -> Scope/6
  Selector9/1 -> Scope/7
  Selector10/1 -> Scope/8
  Selector12/1 -> Scope/9
  Selector11/1 -> Scope/12
  Selector13/1 -> Scope/10
  Selector14/1 -> Scope/11

== system VehicleDynamicsModel/E23/14DOF/14DOF/Subsystem ==
  Info : Inport
  Bus Selector : BusSelector  OutputSignals=InertFrm.FrntAxl.Lft.Disp.X,InertFrm.FrntAxl.Rght.Disp.X,InertFrm.RearAxl.Lft.Disp.X,InertFrm.RearAxl.Rght.Disp.X
  Bus Selector1 : BusSelector  OutputSignals=InertFrm.FrntAxl.Lft.Disp.Y,InertFrm.FrntAxl.Rght.Disp.Y,InertFrm.RearAxl.Lft.Disp.Y,InertFrm.RearAxl.Rght.Disp.Y
  Vector Concatenate : Concatenate  NumInputs=4
  Vector Concatenate1 : Concatenate  NumInputs=4
  XWheel : Outport
  YWheel : Outport  Port=2
  wires:
  Info/1 -> Bus Selector1/1, Bus Selector/1
  Bus Selector/1 -> Vector Concatenate/1  "<X>"
  Bus Selector/2 -> Vector Concatenate/2  "<X>"
  Bus Selector/3 -> Vector Concatenate/3  "<X>"
  Bus Selector/4 -> Vector Concatenate/4  "<X>"
  Vector Concatenate/1 -> XWheel/1
  Bus Selector1/1 -> Vector Concatenate1/1  "<Y>"
  Vector Concatenate1/1 -> YWheel/1
  Bus Selector1/4 -> Vector Concatenate1/4  "<Y>"
  Bus Selector1/2 -> Vector Concatenate1/2  "<Y>"
  Bus Selector1/3 -> Vector Concatenate1/3  "<Y>"

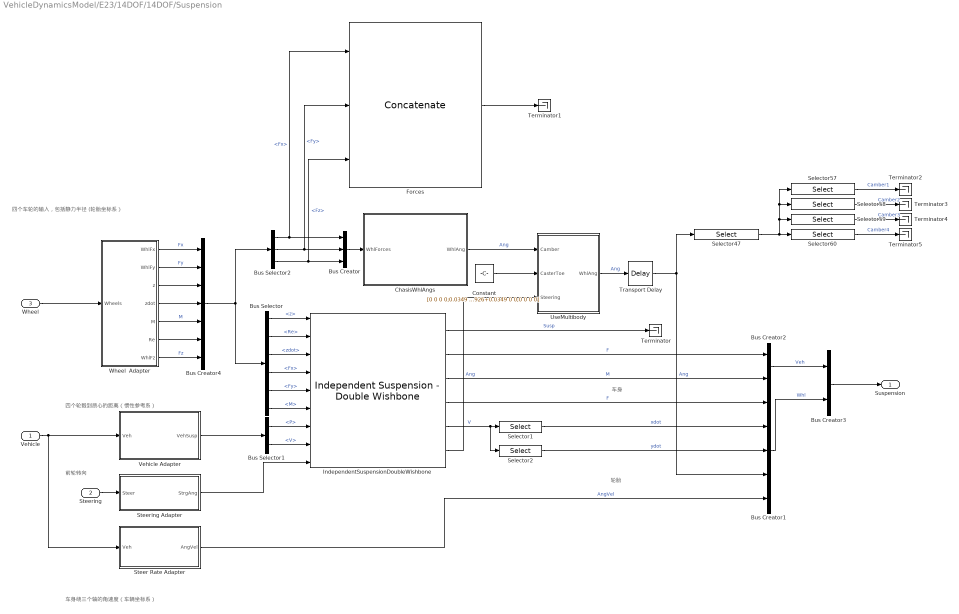
== system VehicleDynamicsModel/E23/14DOF/14DOF/Suspension ==
  note: 车身
  note: 轮胎
  note: 四个轮毂到质心的距离（惯性参考系）
  note: 车身绕三个轴的角速度（车辆坐标系）
  note: 前轮转向
  note: 四个车轮的输入，包括静力半径
      | (轮胎坐标系）
  Vehicle : Inport
  Steering : Inport  Port=2
  Wheel : Inport  Port=3
  Bus Creator : BusCreator  Inputs=3
  Bus Creator1 : BusCreator  Inputs=5
  Bus Creator2 : BusCreator  Inputs=2
  Bus Creator3 : BusCreator  Inputs=2
  Bus Creator4 : BusCreator  Inputs=7
  Bus Selector : BusSelector  OutputSignals=z,Re,zdot,Fx,Fy,M
  Bus Selector1 : BusSelector  OutputSignals=P,V
  Bus Selector2 : BusSelector  OutputSignals=Fx,Fy,Fz
  ChasisWhlAngs : Subsystem
  Constant : Constant  Value=[0 0 0 0;0.0349 3.1415926+0.0349 0 0;0 0 0 0]
  Forces : Concatenate  NumInputs=3  Mode=Multidimensional array
  IndependentSuspensionDoubleWishbone : vehdynlibsuspension/Independent Suspension - Double Wishbone  NumAxl=2  NumTracksByAxl=[2 2]  StrgEnByAxl=[1 0]  AntiSwayEnByAxl=[0 0]  TrackNumVec="[1  2  1  2]"  AxleNumVec="[1  1  2  2]"  SuspTypesByAxle="[1  1]"  SuspImage=suspdw.png  IdealSuspEn=on  IdealSuspAxles="[1  2]"  Kz=Chasis.Kz  F0z=Chasis.F0z  Cz=Chasis.Cz  Hmax=Chasis.Hmax  Toe=0.  RollStrgSlp=0.  ToeStrgSlp=0.  Caster=0.  CasterHslp=0.  CasterStrgSlp=0.  Camber=0.  CamberHslp=0.  CamberStrgSlp=0.  StrgHgtSlp=0.1432  MappedSuspEn=off  MappedSuspAxles="[1  2]"  f_susp_axl_bp=[1 2]  f_susp_dz_bp=[-0.15 -0.14 -0.13 -0.12 -0.11 -0.10 -0.09 -0.08 -0.07 -0.06 -0.05 -0.04 -0.03 -0.02 -0.01 0.00 0.01 0.02 0.03 0.04 0.05 0.06 0.07 0.08 0.09 0.10 0.11 0.12 0.13 0.14 0.15]  f_susp_dzdot_bp=[-0.15 -0.14 -0.13 -0.12 -0.11 -0.10 -0.09 -0.08 -0.07 -0.06 -0.05 -0.04 -0.03 -0.02 -0.01 0.00 0.01 0.02 0.03 0.04 0.05 0.06 0.07 0.08 0.09 0.10 0.11 0.12 0.13 0.14 0.15]  f_susp_fmz=zeros(31,31,61,2,4)  f_susp_geom=zeros(31,61,2,3)  f_susp_strgdelta_bp=[-30,-29,-28,-27,-26,-25,-24,-23,-22,-21,-20,-19,-18,-17,-16,-15,-14,-13,-12,-11,-10,-9,-8,-7,-6,-5,-4,-3,-2,-1,0,1,2,3,4,5,6,7,8,9,10,11,12,13,14,15,16,17,18,19,20,21,22,23,24,25,26,27,28,29,30]  AntiSwayR=0.05  AntiSwayNtrlAng=0.5236  AntiSwayTrsK=8e2
      settings: SourceProductName=Vehicle Dynamics Blockset  SourceProductBaseCode=VE
  Selector1 : Selector  NumberOfDimensions=2  IndexOptions=Index vector (dialog),Select all  Indices=1,1  OutputSizes=1,1
  Selector2 : Selector  NumberOfDimensions=2  IndexOptions=Index vector (dialog),Select all  Indices=2,1  OutputSizes=1,1
  Selector47 : Selector  NumberOfDimensions=2  InputPortWidth=3  IndexOptions=Index vector (dialog),Select all  Indices=1,1  OutputSizes=1,1
  Selector57 : Selector  InputPortWidth=4  IndexOptions=Index vector (dialog)  Indices=1  OutputSizes=1
  Selector58 : Selector  InputPortWidth=4  IndexOptions=Index vector (dialog)  Indices=2  OutputSizes=1
  Selector59 : Selector  InputPortWidth=4  IndexOptions=Index vector (dialog)  Indices=3  OutputSizes=1
  Selector60 : Selector  InputPortWidth=4  IndexOptions=Index vector (dialog)  Indices=4  OutputSizes=1
  Steer Rate Adapter : Subsystem
  Steering Adapter : Subsystem
  Terminator{,1..5} (6 alike) : Terminator
  Transport Delay : TransportDelay  DelayTime=0.1
  UseMultibody : Subsystem  Variant=on  OverrideUsingVariant=Variant
  Vehicle Adapter : Subsystem
  Wheel  Adapter : Subsystem
  Suspension : Outport
  wires:
  IndependentSuspensionDoubleWishbone/5 -> Selector2/1, Selector1/1  "V"
  Wheel  Adapter/4(zdot) -> Bus Creator4/4
  Bus Creator4/1 -> Bus Selector/1, Bus Selector2/1
  IndependentSuspensionDoubleWishbone/3 -> Bus Creator2/2  "M"
  IndependentSuspensionDoubleWishbone/1 -> Terminator/1  "Susp"
  Bus Selector1/1 -> IndependentSuspensionDoubleWishbone/7  "<P>"
  Bus Creator2/1 -> Bus Creator3/1  "Veh"
  Wheel/1 -> Wheel  Adapter/1(Wheels)
  Wheel  Adapter/1(WhlFx) -> Bus Creator4/1  "Fx"
  Wheel  Adapter/2(WhlFy) -> Bus Creator4/2  "Fy"
  Wheel  Adapter/5(M) -> Bus Creator4/5  "M"
  Wheel  Adapter/6(Re) -> Bus Creator4/6
  Selector1/1 -> Bus Creator1/2  "xdot"
  Vehicle/1 -> Steer Rate Adapter/1(Veh), Vehicle Adapter/1(Veh)
  IndependentSuspensionDoubleWishbone/6 -> UseMultibody/3(Steering)  "Ang"
  Bus Selector1/2 -> IndependentSuspensionDoubleWishbone/8  "<V>"
  Bus Creator1/1 -> Bus Creator3/2  "Whl"
  Bus Selector/1 -> IndependentSuspensionDoubleWishbone/1  "<z>"
  Bus Selector/2 -> IndependentSuspensionDoubleWishbone/2  "<Re>"
  Steering Adapter/1(StrgAng) -> IndependentSuspensionDoubleWishbone/9
  Steering/1 -> Steering Adapter/1(Steer)
  Bus Selector/3 -> IndependentSuspensionDoubleWishbone/3  "<zdot>"
  Bus Selector/5 -> IndependentSuspensionDoubleWishbone/5  "<Fy>"
  Steer Rate Adapter/1(AngVel) -> Bus Creator1/5  "AngVel"
  Wheel  Adapter/3(z) -> Bus Creator4/3
  Bus Selector/4 -> IndependentSuspensionDoubleWishbone/4  "<Fx>"
  Selector2/1 -> Bus Creator1/3  "ydot"
  Bus Creator3/1 -> Suspension/1
  Vehicle Adapter/1(VehSusp) -> Bus Selector1/1
  Bus Selector/6 -> IndependentSuspensionDoubleWishbone/6  "<M>"
  Wheel  Adapter/7(WhlFz) -> Bus Creator4/7  "Fz"
  Bus Selector2/1 -> Bus Creator/1, Forces/1  "<Fx>"
  Bus Selector2/2 -> Forces/2, Bus Creator/2  "<Fy>"
  Bus Selector2/3 -> Forces/3, Bus Creator/3  "<Fz>"
  Bus Creator/1 -> ChasisWhlAngs/1(WhlForces)
  Selector60/1 -> Terminator5/1  "Camber4"
  Selector59/1 -> Terminator4/1  "Camber3"
  Selector58/1 -> Terminator3/1  "Camber2"
  Selector57/1 -> Terminator2/1  "Camber1"
  Selector47/1 -> Selector57/1, Selector58/1, Selector59/1, Selector60/1
  IndependentSuspensionDoubleWishbone/4 -> Bus Creator1/1  "F"
  IndependentSuspensionDoubleWishbone/2 -> Bus Creator2/1  "F"
  Forces/1 -> Terminator1/1
  ChasisWhlAngs/1(WhlAng) -> UseMultibody/1(Camber)  "Ang"
  UseMultibody/1(WhlAng) -> Transport Delay/1  "Ang"
  Constant/1 -> UseMultibody/2(CasterToe)
  Transport Delay/1 -> Selector47/1, Bus Creator1/4  "Ang"

== system VehicleDynamicsModel/E23/14DOF/14DOF/Tires&Wheels ==
  note: 内倾角
  note: 前束角
  note: 附着系数
  note: 路面输入
  Suspension : Inport
  AxleTorque : Inport  Port=2
  BrakerPress : Inport  Port=3
  GndInput : Inport  Port=4
  Friction : Inport  Port=5
  Bus Selector : BusSelector  OutputSignals=Whl.Ang,Whl.F,Whl.AngVel,Whl.xdot,Whl.ydot
  Cont LPF1 : autolibutils/Cont LPF  wc=100*2*pi  aMode=2
      settings: SourceProductName=Powertrain Blockset  SourceProductBaseCode=PW
  Cont LPF2 : autolibutils/Cont LPF  wc=100*2*pi  aMode=2
      settings: SourceProductName=Powertrain Blockset  SourceProductBaseCode=PW
  Matrix Concatenate : Concatenate  NumInputs=3  Mode=Multidimensional array
  Reshape : Reshape
  Reshape1 : Reshape
  Saturation : Saturate  UpperLimit=Inf  LowerLimit=-10*9.81*2000
  Selector : Selector  NumberOfDimensions=2  InputPortWidth=3  IndexOptions=Index vector (dialog),Select all  Indices=3,1  OutputSizes=1,1
  Selector1 : Selector  NumberOfDimensions=2  InputPortWidth=3  IndexOptions=Index vector (dialog),Select all  Indices=1,1  OutputSizes=1,1
  Selector2 : Selector  NumberOfDimensions=2  InputPortWidth=3  IndexOptions=Index vector (dialog),Select all  Indices=[3],1  OutputSizes=1,1
  Selector3 : Selector  NumberOfDimensions=2  InputPortWidth=3  IndexOptions=Index vector (dialog),Select all  Indices=[3],1  OutputSizes=1,1
  Terminator{,1..4} (5 alike) : Terminator
  VDBS : Subsystem
  Wheels : Outport
  wires:
  VDBS/2(FL) -> Terminator/1
  VDBS/5(SuspWhlPz) -> Terminator3/1
  VDBS/4(FR) -> Terminator2/1
  VDBS/3(WhlOmega) -> Terminator1/1
  VDBS/1(Wheels) -> Wheels/1  "Wheels"
  Suspension/1 -> Bus Selector/1
  Bus Selector/1 -> Cont LPF1/1  "<Ang>"
  Cont LPF1/1 -> Selector1/1, Selector/1
  Selector/1 -> VDBS/1(WheelAng)
  Selector1/1 -> VDBS/2(CamberAng)
  Bus Selector/2 -> Selector2/1  "<F>"
  Selector2/1 -> Reshape/1
  Reshape/1 -> Cont LPF2/1
  Cont LPF2/1 -> Saturation/1
  Saturation/1 -> VDBS/5(Fz)
  BrakerPress/1 -> VDBS/4(BrkPrs)
  AxleTorque/1 -> VDBS/3(AxleTrq)
  Bus Selector/3 -> Selector3/1  "<AngVel>"
  Selector3/1 -> Reshape1/1
  Reshape1/1 -> VDBS/6(r)
  Bus Selector/4 -> Matrix Concatenate/1  "<xdot>"
  Bus Selector/5 -> Matrix Concatenate/2  "<ydot>"
  Matrix Concatenate/1 -> VDBS/7(VehVel)
  GndInput/1 -> VDBS/8(GroundLevel)
  Friction/1 -> VDBS/9(Friction)
  VDBS/6(SuspWhlVz) -> Matrix Concatenate/3  "zdot"
  VDBS/7(SteerTrq) -> Terminator4/1

== system VehicleDynamicsModel/E23/PowerTrain/DriveTrain/DriveLine ==
  SteerCmd : Inport
  AxleTrqCmd : Inport  Port=2
  BrkPrsCmd : Inport  Port=3
  BrkPrs : Subsystem
  Ground : Ground
  Kinematic Steering : vehdynlibsteering/Kinematic Steering  StrgType=Ackerman  StrgRatioType=Constant  Loc=Front  NrmlFctr=0.01  TrckWdth=VEH.TrackWidth(1)  WhlBase=VEH.FrontAxlePositionfromCG+VEH.RearAxlePositionfromCG  Db=0  StrgRng=pi/2  StrgAngBpts="[-6.2832   -5.0265   -3.7699   -2.5133   -1.2566         0    1.2566    2.5133    3.7699    5.0265    6.2832]"  StrgRatioTbl=|  StrgRatio=1  StrgArmLngth=0.1  RckCsLngth=0.5  TieRodLngth=0.248  D=0.2  PnnRadius=0.0057  PnnRadiusTbl="[0.0055    0.0055    0.0056    0.0057    0.0058    0.0057    0.0057    0.0057    0.0056    0.0055    0.0055]"  RodLngth=0.1  ParaArmLngth=0.9  aMode=2
      | [13.5000   13.3750   13.2500   13.1250   13.0000   13.0000   13.0000   13.1250   13.2500   13.3750   13.5000
      | ]
      settings: SourceProductName=Vehicle Dynamics Blockset
  Terminator : Terminator
  Vector Concatenate : Concatenate
  Vector Concatenate1 : Concatenate
  Vector Concatenate2 : Concatenate
  AxleTrq : Outport
  BrakePressure : Outport  Port=2
  WhlAng : Outport  Port=3
  wires:
  Vector Concatenate1/1 -> Vector Concatenate/1
  Kinematic Steering/3 -> Vector Concatenate1/2
  BrkPrsCmd/1 -> BrkPrs/1(BrkPrsCmd)
  AxleTrqCmd/1 -> AxleTrq/1
  Vector Concatenate2/1 -> Vector Concatenate/2
  Ground/1 -> Vector Concatenate2/1, Vector Concatenate2/2
  Kinematic Steering/2 -> Vector Concatenate1/1
  Kinematic Steering/1 -> Terminator/1
  Vector Concatenate/1 -> WhlAng/1
  SteerCmd/1 -> Kinematic Steering/1
  BrkPrs/1(BrkPrs) -> BrakePressure/1

== system VehicleDynamicsModel/E23/PowerTrain/DriveTrain/MotorTrq2AxleTrq ==
  MotorRL : Inport
  MotorRR : Inport  Port=2
  Gain3 : Gain  Gain=GearRatio
  Gain4 : Gain  Gain=GearRatio
  Ground : Ground
  Vector Concatenate : Concatenate
  Vector Concatenate1 : Concatenate
  Vector Concatenate2 : Concatenate
  AxleTrq : Outport
  wires:
  MotorRR/1 -> Gain3/1
  Gain4/1 -> Vector Concatenate/1
  Ground/1 -> Vector Concatenate1/1, Vector Concatenate1/2
  Gain3/1 -> Vector Concatenate/2
  MotorRL/1 -> Gain4/1
  Vector Concatenate2/1 -> AxleTrq/1
  Vector Concatenate1/1 -> Vector Concatenate2/1
  Vector Concatenate/1 -> Vector Concatenate2/2

== system VehicleDynamicsModel/E23/PowerTrain/PowerTrain/MotorRL ==
  TrqCmd : Inport
  MtrSpd : Inport  Port=2
  MtrVol : Inport  Port=3
  Motor : Subsystem
      mask Display: image('Motor.jpg');
  MechPwr : Outport
  Efficiency : Outport  Port=2
  MtrTrq : Outport  Port=3
  wires:
  Motor/3(MtrTrq) -> MtrTrq/1  "MtrTrq"
  TrqCmd/1 -> Motor/1(TrqCmd)
  Motor/2(Efficiency) -> Efficiency/1  "Efficiency"
  Motor/1(MechPwr) -> MechPwr/1  "MechPwr"
  MtrSpd/1 -> Motor/3(MtrSpd)
  MtrVol/1 -> Motor/2(BattVolt)

== system VehicleDynamicsModel/E23/PowerTrain/PowerTrain/MotorRR ==
  TrqCmd : Inport
  MtrSpd : Inport  Port=2
  MtrVol : Inport  Port=3
  Motor : Subsystem
      mask Display: image('Motor.jpg');
  MechPwr : Outport
  Efficiency : Outport  Port=2
  MtrTrq : Outport  Port=3
  wires:
  Motor/3(MtrTrq) -> MtrTrq/1  "MtrTrq"
  TrqCmd/1 -> Motor/1(TrqCmd)
  Motor/2(Efficiency) -> Efficiency/1  "Efficiency"
  Motor/1(MechPwr) -> MechPwr/1  "MechPwr"
  MtrSpd/1 -> Motor/3(MtrSpd)
  MtrVol/1 -> Motor/2(BattVolt)

== system VehicleDynamicsModel/E23/14DOF/14DOF/Suspension/ChasisWhlAngs ==
  WhlForces : Inport
  Bus Selector2 : BusSelector  OutputSignals=Fx,Fy,Fz
  Variant Subsystem : Subsystem  Variant=on  OverrideUsingVariant=Variant1
  WhlAng : Outport
  wires:
  WhlForces/1 -> Bus Selector2/1
  Bus Selector2/1 -> Variant Subsystem/1(FxR)  "<Fx>"
  Bus Selector2/2 -> Variant Subsystem/2(FyR)  "<Fy>"
  Bus Selector2/3 -> Variant Subsystem/3(FzR)  "<Fz>"
  Variant Subsystem/1(WhlAng) -> WhlAng/1

== system VehicleDynamicsModel/E23/14DOF/14DOF/Suspension/Steer Rate Adapter ==
  Veh : Inport
  Add : Sum
  Bus Selector3 : BusSelector  OutputSignals=BdyFrm.Cg.AngVel.r
  Constant : Constant  Value=zeros(1,4)
  Matrix Concatenate : Concatenate  NumInputs=3  Mode=Multidimensional array
  Matrix Concatenate1 : Concatenate  NumInputs=3  Mode=Multidimensional array
  Reshape2 : Reshape  OutputDimensionality=Row vector (2-D)
  Reshape3 : Reshape  OutputDimensionality=Row vector (2-D)
  Reshape4 : Reshape  OutputDimensionality=Row vector (2-D)
  Selector3 : Selector  InputPortWidth=1  IndexOptions=Index vector (dialog)  Indices=[1 1 1 1]  OutputSizes=1
  SteerRates : Constant  Value=zeros(1,4)
  AngVel : Outport
  wires:
  Reshape2/1 -> Matrix Concatenate1/1, Matrix Concatenate1/2, Matrix Concatenate1/3
  Constant/1 -> Reshape3/1
  Selector3/1 -> Reshape4/1
  Bus Selector3/1 -> Selector3/1  "<r>"
  Matrix Concatenate/1 -> Add/2
  SteerRates/1 -> Reshape2/1
  Reshape4/1 -> Matrix Concatenate/3
  Reshape3/1 -> Matrix Concatenate/1, Matrix Concatenate/2
  Matrix Concatenate1/1 -> Add/1
  Veh/1 -> Bus Selector3/1
  Add/1 -> AngVel/1  "AngVel"

== system VehicleDynamicsModel/E23/14DOF/14DOF/Suspension/Steering Adapter ==
  Steer : Inport
  Reshape1 : Reshape  OutputDimensionality=Row vector (2-D)
  Selector : Selector  IndexOptions=Index vector (dialog)  Indices=[1 2]  OutputSizes=1
  StrgAng : Outport
  wires:
  Reshape1/1 -> StrgAng/1
  Steer/1 -> Selector/1
  Selector/1 -> Reshape1/1

== system VehicleDynamicsModel/E23/14DOF/14DOF/Suspension/UseMultibody ==
  note: 1) Add Subsystem or Model blocks as valid variant choices.
      | 2) You cannot connect blocks at this level. At simulation, connectivity is automatically
      | determined, based on the active variant and port name matching.
  Camber : Inport
  CasterToe : Inport  Port=2
  Steering : Inport  Port=3
  No : Subsystem  VariantControl=Variant1
  Yes : Subsystem  VariantControl=Variant
  WhlAng : Outport

== system VehicleDynamicsModel/E23/14DOF/14DOF/Suspension/Vehicle Adapter ==
  Veh : Inport
  Bus Creator3 : BusCreator  Inputs=2
  Bus Selector1 : BusSelector  OutputSignals=InertFrm.FrntAxl.Lft.Disp.X,InertFrm.FrntAxl.Lft.Disp.Y,InertFrm.FrntAxl.Lft.Disp.Z,InertFrm.FrntAxl.Rght.Disp.X,InertFrm.FrntAxl.Rght.Disp.Y,InertFrm.FrntAxl.Rght.Disp.Z,InertFrm.RearAxl.Lft.Disp.X,InertFrm.RearAxl.Lft.Disp.Y,InertFrm.RearAxl.Lft.Disp.Z,InertFrm.RearAxl.Rght.Disp.X,InertFrm.RearAxl.Rght.Disp.Y,InertFrm.RearAxl.Rght.Disp.Z
  Bus Selector2 : BusSelector  OutputSignals=BdyFrm.FrntAxl.Lft.Vel.xdot,BdyFrm.FrntAxl.Lft.Vel.ydot,BdyFrm.FrntAxl.Lft.Vel.zdot,BdyFrm.FrntAxl.Rght.Vel.xdot,BdyFrm.FrntAxl.Rght.Vel.ydot,BdyFrm.FrntAxl.Rght.Vel.zdot,BdyFrm.RearAxl.Lft.Vel.xdot,BdyFrm.RearAxl.Lft.Vel.ydot,BdyFrm.RearAxl.Lft.Vel.zdot,BdyFrm.RearAxl.Rght.Vel.xdot,BdyFrm.RearAxl.Rght.Vel.ydot,BdyFrm.RearAxl.Rght.Vel.zdot
  Inertial Frame CG to Axle Offset : Constant  Value=[zeros(2,4);VEH.HeightCG*ones(1,4)]
  Mux1 : Mux  Inputs=12
  Mux2 : Mux  Inputs=12
  Reshape1 : Reshape  OutputDimensionality=Customize  OutputDimensions=[3,4]
  Reshape2 : Reshape  OutputDimensionality=Customize  OutputDimensions=[3,4]
  Sum : Sum  Inputs=|+-
  VehSusp : Outport
  wires:
  Reshape2/1 -> Bus Creator3/2  "V"
  Bus Creator3/1 -> VehSusp/1  "Veh"
  Bus Selector1/1 -> Mux2/1  "<X>"
  Bus Selector1/2 -> Mux2/2  "<Y>"
  Bus Selector1/3 -> Mux2/3  "<Z>"
  Bus Selector1/4 -> Mux2/4  "<X>"
  Bus Selector1/5 -> Mux2/5  "<Y>"
  Bus Selector1/6 -> Mux2/6  "<Z>"
  Bus Selector1/7 -> Mux2/7  "<X>"
  Bus Selector1/8 -> Mux2/8  "<Y>"
  Bus Selector1/9 -> Mux2/9  "<Z>"
  Bus Selector1/10 -> Mux2/10  "<X>"
  Bus Selector1/11 -> Mux2/11  "<Y>"
  Bus Selector1/12 -> Mux2/12  "<Z>"
  Bus Selector2/1 -> Mux1/1  "<xdot>"
  Bus Selector2/2 -> Mux1/2  "<ydot>"
  Bus Selector2/3 -> Mux1/3  "<zdot>"
  Bus Selector2/4 -> Mux1/4  "<xdot>"
  Bus Selector2/5 -> Mux1/5  "<ydot>"
  Bus Selector2/6 -> Mux1/6  "<zdot>"
  Bus Selector2/7 -> Mux1/7  "<xdot>"
  Bus Selector2/8 -> Mux1/8  "<ydot>"
  Bus Selector2/9 -> Mux1/9  "<zdot>"
  Bus Selector2/10 -> Mux1/10  "<xdot>"
  Bus Selector2/11 -> Mux1/11  "<ydot>"
  Bus Selector2/12 -> Mux1/12  "<zdot>"
  Mux1/1 -> Reshape2/1
  Inertial Frame CG to Axle Offset/1 -> Sum/2
  Sum/1 -> Bus Creator3/1  "P"
  Veh/1 -> Bus Selector2/1, Bus Selector1/1
  Mux2/1 -> Reshape1/1
  Reshape1/1 -> Sum/1

== system VehicleDynamicsModel/E23/14DOF/14DOF/Suspension/Wheel  Adapter ==
  Wheels : Inport
  Bus Selector : BusSelector  OutputSignals=TireFrame.Fx,TireFrame.Fy,TireFrame.Fz
  Bus Selector1 : BusSelector  OutputSignals=TireFrame.Re
  Bus Selector2 : BusSelector  OutputSignals=TireFrame.Mx,TireFrame.My,TireFrame.Mz
  Bus Selector3 : BusSelector  OutputSignals=TireFrame.z,TireFrame.zdot
  Matrix Concatenate : Concatenate  NumInputs=3  Mode=Multidimensional array
  Reshape{,1..8} (9 alike) : Reshape  OutputDimensionality=Row vector (2-D)
  WhlFx : Outport
  WhlFy : Outport  Port=2
  z : Outport  Port=3
  zdot : Outport  Port=4
  M : Outport  Port=5
  Re : Outport  Port=6
  WhlFz : Outport  Port=7
  wires:
  Reshape7/1 -> WhlFy/1
  Reshape6/1 -> WhlFx/1
  Bus Selector/1 -> Reshape6/1  "<Fx>"
  Bus Selector/2 -> Reshape7/1  "<Fy>"
  Bus Selector3/1 -> Reshape/1  "<z>"
  Wheels/1 -> Bus Selector1/1, Bus Selector2/1, Bus Selector3/1, Bus Selector/1
  Bus Selector3/2 -> Reshape2/1  "<zdot>"
  Reshape2/1 -> zdot/1  "zdot"
  Bus Selector1/1 -> Reshape1/1  "<Re>"
  Reshape1/1 -> Re/1  "Re"
  Bus Selector2/1 -> Reshape3/1  "<Mx>"
  Bus Selector2/2 -> Reshape4/1  "<My>"
  Bus Selector2/3 -> Reshape5/1  "<Mz>"
  Reshape3/1 -> Matrix Concatenate/1
  Reshape4/1 -> Matrix Concatenate/2
  Reshape5/1 -> Matrix Concatenate/3
  Matrix Concatenate/1 -> M/1  "M"
  Reshape/1 -> z/1  "z"
  Bus Selector/3 -> Reshape8/1  "<Fz>"
  Reshape8/1 -> WhlFz/1
